simulink model "ProgettoMixSen"  (R2021a)
settings: Solver=VariableStepAuto  StartTime=0.0  StopTime=30  RelTol=1e-3
undefined symbols (not defined in the file): A, Ak, B, Bk, Ck, Dk, Qt, Rt
libraries: simulink x3
settings Model: Creator=a15le  LastModifiedBy=a15le

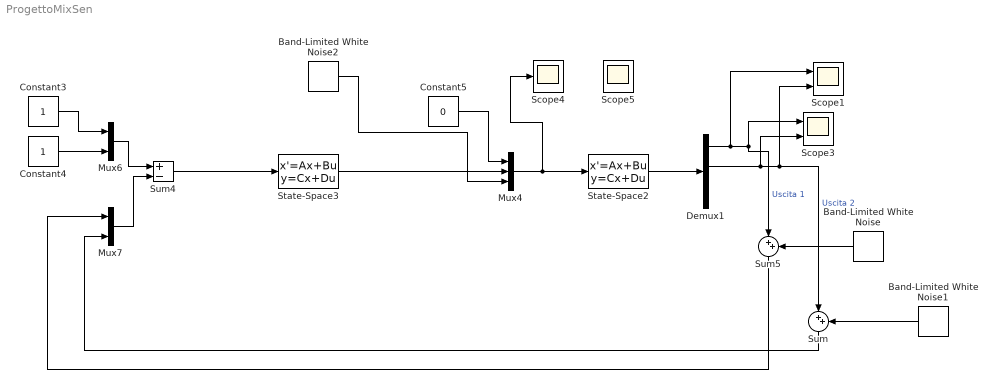
== system ProgettoMixSen ==
  Band-Limited White Noise : simulink/Sources/Band-Limited White Noise  Cov=diag(Rt)*1e-3*0  Ts=1e-3  seed=[23341]
  Band-Limited White Noise1 : simulink/Sources/Band-Limited White Noise  Cov=diag(Rt)*1e-3*0  Ts=1e-3  seed=[23341]
  Band-Limited White Noise2 : simulink/Sources/Band-Limited White Noise  Cov=diag(Qt)*1e-3*0  Ts=1e-3  seed=[23341]
  Constant3 : Constant
  Constant4 : Constant
  Constant5 : Constant  Value=0
  Demux1 : Demux  Outputs=6
  Mux4 : Mux  Inputs=3
  Mux6 : Mux  Inputs=2
  Mux7 : Mux  Inputs=2
  Scope1 : Scope  NumInputPorts=2
  Scope3 : Scope  NumInputPorts=2
  Scope4 : Scope
  Scope5 : Scope
  State-Space2 : StateSpace  A=A  B=[B eye(6)]  C=eye(6)  D=zeros(6,9)  InitialCondition=0  ParameterTunability=Optimized
  State-Space3 : StateSpace  A=Ak  B=Bk  C=Ck  D=Dk  InitialCondition=0
  Sum : Sum  Inputs=|++
  Sum4 : Sum  Inputs=+-
  Sum5 : Sum  Inputs=|++
  wires:
  Sum5/1 -> Mux7/1
  Mux6/1 -> Sum4/1
  Constant3/1 -> Mux6/1
  Constant5/1 -> Mux4/1
  Sum4/1 -> State-Space3/1
  Band-Limited White Noise2/1 -> Mux4/3
  Mux4/1 -> Scope4/1, State-Space2/1
  Constant4/1 -> Mux6/2
  State-Space2/1 -> Demux1/1
  Mux7/1 -> Sum4/2
  Band-Limited White Noise/1 -> Sum5/2
  State-Space3/1 -> Mux4/2
  Band-Limited White Noise1/1 -> Sum/2
  Sum/1 -> Mux7/2
  Demux1/1 -> Scope1/1, Sum5/1, Scope3/1  "Uscita 1"
  Demux1/3 -> Scope1/2, Sum/1, Scope3/2  "Uscita 2"
